simulink model "sistem_3"  (R2025b)
settings: Solver=VariableStepAuto  StartTime=0.0  StopTime=150  RelTol=1e-3
values from neighbouring files (symbols this model uses):
  a1 = 0.0350211586167    [sistem_3.mat]
  a2 = 0.0039    [sistem_3.mat]
  a3 = 0.000137177878301    [sistem_3.mat]
  a4 = 2.32190281628e-09    [sistem_3.mat]
  a5 = 0.496133080403    [sistem_3.mat]
  a6 = 1.7e-06    [sistem_3.mat]
settings Model: Creator=RIZKI  LastModifiedBy=RIZKI

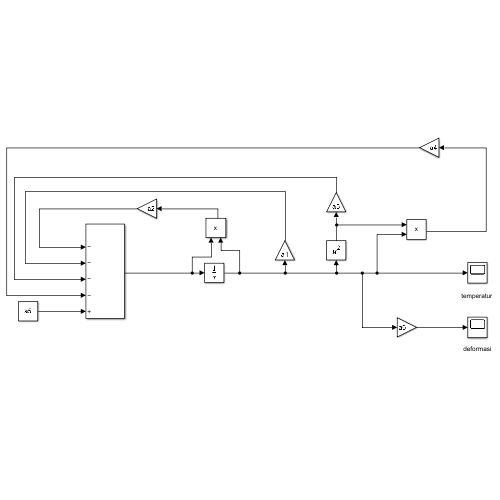
[thumbnail: Simulink's stored preview of the top-level diagram]
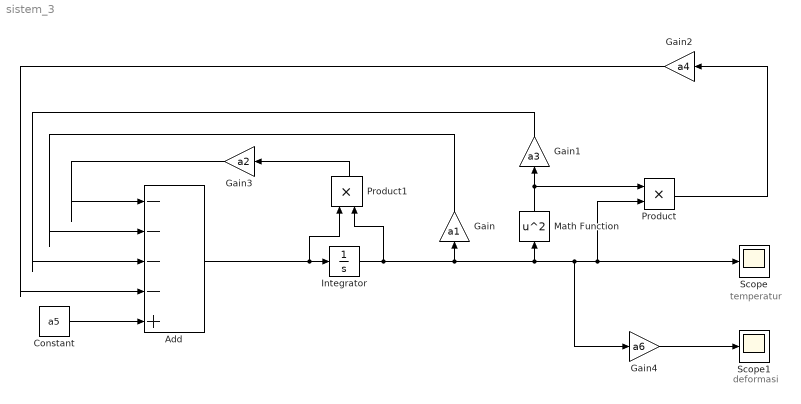
== system sistem_3 ==
  note: deformasi
  note: temperatur
  Add : Sum  Inputs=|----+
  Constant : Constant  Value=a5
  Gain : Gain  Gain=a1
  Gain1 : Gain  Gain=a3
  Gain2 : Gain  Gain=a4
  Gain3 : Gain  Gain=a2
  Gain4 : Gain  Gain=a6
  Integrator : Integrator
  Math Function : Math  Operator=square
  Product : Product
  Product1 : Product
  Scope : Scope
      settings: ActiveDisplayYMinimum=-1.6754046537175176  ActiveDisplayYMaximum=15.078641883457662
  Scope1 : Scope
      settings: ActiveDisplayYMinimum=-2.8481879113197803E-6  ActiveDisplayYMaximum=2.5633691201878028E-5
  wires:
  Constant/1 -> Add/5
  Integrator/1 -> Math Function/1, Gain4/1, Product/2, Scope/1, Gain/1, Product1/2
  Gain/1 -> Add/2
  Math Function/1 -> Product/1, Gain1/1
  Gain1/1 -> Add/3
  Product/1 -> Gain2/1
  Gain2/1 -> Add/4
  Add/1 -> Product1/1, Integrator/1
  Product1/1 -> Gain3/1
  Gain3/1 -> Add/1
  Gain4/1 -> Scope1/1
